simulink model "motor_test"  (R2015a)
settings: Solver=ode3  StartTime=0.0  StopTime=10  RelTol=1e-3
undefined symbols (not defined in the file or in its folder): MIO, National_Instruments, PCI
libraries: sldrtlib x2, simulink x1
settings Model: SimulationMode=external  ExtModeTrigDuration=200000  Creator=Alunos  LastModifiedBy=Alunos
settings HardwareCC: ProdIntDivRoundTo=Zero  ProdEndianess=LittleEndian  ProdHWDeviceType=Intel->x86/Pentium  TargetIntDivRoundTo=Zero  TargetEndianess=LittleEndian  TargetHWDeviceType=Intel->x86/Pentium
settings RTWCC: SystemTargetFile=rtwin.tlc  TemplateMakefile=rtwin.tmf  Description=Simulink Desktop Real-Time  RTWCompilerOptimization=on
settings CodeAppCC: MaxIdLength=95
settings RTWinTargetCC: TargetPreCompLibLocation=C:\Program Files\MATLAB\R2015a\toolbox\sldrt\lib\win32

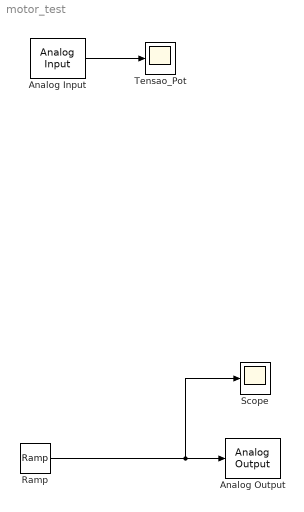
== system motor_test ==
  Analog Input : sldrtlib/Analog Input  SampleTime=0.001  MaxMissedTicks=10  ShowMissedTicks=off  YieldWhenWaiting=off  DrvName=National_Instruments/PCI-MIO-16E-4  DrvAddress=4294967295  DrvOptions=[0 0 0 0 0 0]  Channels=[1 2]  RangeMode=1  VoltRange=1  DataType=1
      settings: AttributesFormatString=National Instruments\nPCI-MIO-16E-4 [auto]
  Analog Output : sldrtlib/Analog Output  SampleTime=0.001  MaxMissedTicks=10  ShowMissedTicks=off  YieldWhenWaiting=off  DrvName=National_Instruments/PCI-MIO-16E-4  DrvAddress=4294967295  DrvOptions=[0 0 0 0 0 0]  Channels=1  RangeMode=1  VoltRange=1  InitialValue=0  FinalValue=0
      settings: AttributesFormatString=National Instruments\nPCI-MIO-16E-4 [auto]
  Ramp : simulink/Sources/Ramp  slope=0.1  start=1  X0=0
  Scope : Scope
      settings: TickLabels=on  SaveName=input  SampleInput=on  SampleTime=0.001
  Tensao_Pot : Scope
      settings: TickLabels=on  YMin=-5.5  YMax=5.5  SaveName=tensao_pot  SampleInput=on  SampleTime=0.001
  wires:
  Analog Input/1 -> Tensao_Pot/1
  Ramp/1 -> Scope/1, Analog Output/1
